simulink model "K_opt"  (R2023b)
settings: Solver=VariableStepAuto  StartTime=0.0  StopTime=10.0  RelTol=1e-3
settings Model: Creator=54238  LastModifiedBy=54238
settings RTWCC: GPUComputeCapability=5.0

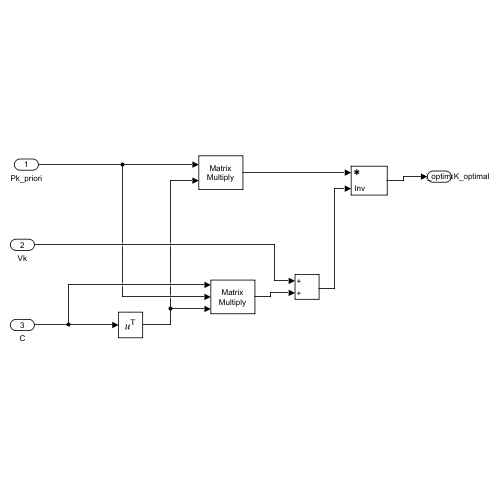
[thumbnail: Simulink's stored preview of the top-level diagram]
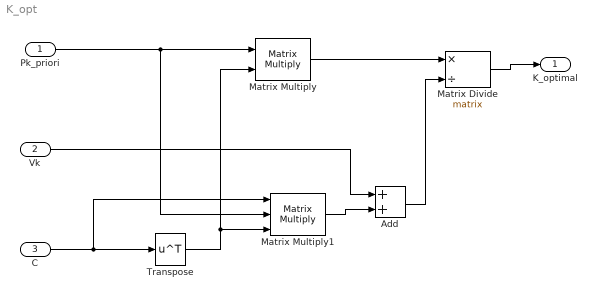
== system K_opt ==
  Pk_priori : Inport
  Vk : Inport  Port=2
  C : Inport  Port=3
  Add : Sum
  Matrix Divide : Product  Inputs=*/  Multiplication=Matrix(*)
  Matrix Multiply : Product  Multiplication=Matrix(*)
  Matrix Multiply1 : Product  Inputs=3  Multiplication=Matrix(*)
  Transpose : Math  Operator=transpose
  K_optimal : Outport  SignalName=K_optimal
  wires:
  C/1 -> Matrix Multiply1/1, Transpose/1
  Pk_priori/1 -> Matrix Multiply1/2, Matrix Multiply/1
  Transpose/1 -> Matrix Multiply1/3, Matrix Multiply/2
  Matrix Multiply1/1 -> Add/2
  Vk/1 -> Add/1
  Add/1 -> Matrix Divide/2
  Matrix Multiply/1 -> Matrix Divide/1
  Matrix Divide/1 -> K_optimal/1
